simulink model "input_signal_test"  (R2013a)
settings: Solver=VariableStepDiscrete  StartTime=0.0  StopTime=10.0  MaxStep=0.01  RelTol=1e-3
undefined symbols (not defined in the file or in its folder): da, dp, ds, r
libraries: cstblocks x4
settings Model: Creator=Vittorio  LastModifiedBy=s171105
settings OptimizationCC: ExpressionDepthLimit=2147483647
settings DebuggingCC: StrictBusMsg=Warning
settings GRTTargetCC: CombineOutputUpdateFcns=off  GRTInterface=on

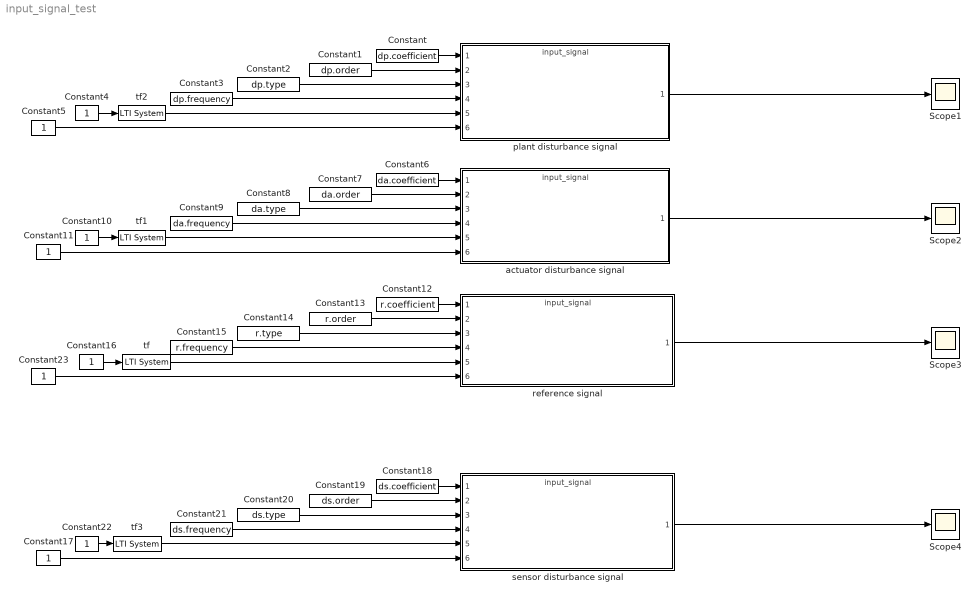
== system input_signal_test ==
  Constant : Constant  Value=dp.coefficient
  Constant1 : Constant  Value=dp.order
  Constant{4..5,10..11,16..17,22..23} (8 alike) : Constant
  Constant12 : Constant  Value=r.coefficient
  Constant13 : Constant  Value=r.order
  Constant14 : Constant  Value=r.type
  Constant15 : Constant  Value=r.frequency
  Constant18 : Constant  Value=ds.coefficient
  Constant19 : Constant  Value=ds.order
  Constant2 : Constant  Value=dp.type
  Constant20 : Constant  Value=ds.type
  Constant21 : Constant  Value=ds.frequency
  Constant3 : Constant  Value=dp.frequency
  Constant6 : Constant  Value=da.coefficient
  Constant7 : Constant  Value=da.order
  Constant8 : Constant  Value=da.type
  Constant9 : Constant  Value=da.frequency
  Scope{1..4} (4 alike) : Scope
      Scope3 settings: SaveName=ScopeData2
      Scope4 settings: SaveName=ScopeData3
  actuator disturbance signal : ModelReference  ModelNameDialog=input_signal  ModelReferenceVersion=1.18  CopyOfModelName=input_signal  DefaultDataLogging=off
  plant disturbance signal : ModelReference  ModelNameDialog=input_signal  ModelReferenceVersion=1.18  CopyOfModelName=input_signal  DefaultDataLogging=off
  reference signal : ModelReference  ModelNameDialog=input_signal  ModelReferenceVersion=1.18  CopyOfModelName=input_signal  DefaultDataLogging=off
  sensor disturbance signal : ModelReference  ModelNameDialog=input_signal  ModelReferenceVersion=1.18  CopyOfModelName=input_signal  DefaultDataLogging=off
  tf : cstblocks/LTI System  sys=r.tf  IC=[]
  tf1 : cstblocks/LTI System  sys=da.tf  IC=[]
  tf2 : cstblocks/LTI System  sys=dp.tf  IC=[]
  tf3 : cstblocks/LTI System  sys=ds.tf  IC=[]
  wires:
  Constant/1 -> plant disturbance signal/1
  Constant1/1 -> plant disturbance signal/2
  Constant2/1 -> plant disturbance signal/3
  Constant3/1 -> plant disturbance signal/4
  tf2/1 -> plant disturbance signal/5
  Constant6/1 -> actuator disturbance signal/1
  Constant7/1 -> actuator disturbance signal/2
  Constant8/1 -> actuator disturbance signal/3
  Constant9/1 -> actuator disturbance signal/4
  tf1/1 -> actuator disturbance signal/5
  Constant11/1 -> actuator disturbance signal/6
  Constant12/1 -> reference signal/1
  Constant13/1 -> reference signal/2
  Constant14/1 -> reference signal/3
  Constant15/1 -> reference signal/4
  tf/1 -> reference signal/5
  Constant23/1 -> reference signal/6
  Constant18/1 -> sensor disturbance signal/1
  Constant19/1 -> sensor disturbance signal/2
  Constant20/1 -> sensor disturbance signal/3
  Constant21/1 -> sensor disturbance signal/4
  tf3/1 -> sensor disturbance signal/5
  Constant17/1 -> sensor disturbance signal/6
  Constant16/1 -> tf/1
  Constant10/1 -> tf1/1
  Constant4/1 -> tf2/1
  Constant22/1 -> tf3/1
  Constant5/1 -> plant disturbance signal/6
  plant disturbance signal/1 -> Scope1/1
  actuator disturbance signal/1 -> Scope2/1
  reference signal/1 -> Scope3/1
  sensor disturbance signal/1 -> Scope4/1
